simulink model "BMS_model_balancing"  (R2025b)
settings: Solver=FixedStepDiscrete  StartTime=0.0  StopTime=10  RelTol=1e-3
undefined symbols (not defined in the file): balanceResis, BalThreshold, chargeCurrent, currentLim, dischargeCurrent, initialSOC, stepTime, tempLim, Ts
libraries: fl_lib x128, nesl_utility x105, ee_lib x24, batteryecm_lib x24, simulink x5, BatteryBalancing x2, BatteryCurrentManagement x1
(part 1 of 5)
settings Model: Creator=Kevin  LastModifiedBy=kevpc
settings DataIOCC: ExternalInput=test_temp.getElement('Temp 1'),test_temp.getElement('Temp 2')  LoadExternalInput=on
settings OptimizationCC: DefaultParameterBehavior=Inlined  EnhancedBackFolding=on  PassReuseOutputArgsAs=Individual arguments  ZeroExternalMemoryAtStartup=off  ZeroInternalMemoryAtStartup=off  OptimizeBlockOrder=speed  DifferentSizesBufferReuse=on  OptimizationCustomize=off  EfficientTunableParamExpr=on
settings DebuggingCC: SolverPrmCheckMsg=warning  ParameterTunabilityLossMsg=error  StateNameClashWarn=warning
settings HardwareCC: ProdBitPerInt=16.0  ProdBitPerPointer=16.0  ProdBitPerSizeT=16.0  ProdBitPerPtrDiffT=16.0  ProdLargestAtomicFloat=None  ProdWordSize=16.0  ProdHWDeviceType=STMicroelectronics->ST10/Super10
settings SFSimCC: MATLABDynamicMemAlloc=off  SimTargetLang=C++  SimDLTargetLibrary=mkl-dnn
settings RTWCC: SystemTargetFile=ert.tlc  TemplateMakefile=ert_default_tmf  BuildConfiguration=Faster Runs  PortableWordSizes=on  DataTypeReplacement=CDataTypesFixedWidth  TargetLang=C++  GPUComputeCapability=3.5  Description=Embedded Coder
settings CodeAppCC: ForceParamTrailComments=on  IgnoreCustomStorageClasses=off  OperatorAnnotations=on  SimulinkDataObjDesc=on  SFDataObjDesc=on  MATLABFcnDesc=on  InsertBlockDesc=on  StateflowObjectComments=on  InlinedPrmAccess=Macros
settings ERTTargetCC: RootIOFormat=Structure reference  ERTCustomFileTemplate=example_file_process.tlc  ERTFilePackagingFormat=Compact  SuppressUnreachableDefaultCases=off  IndentSize=4  MaxIdInt64=INT64_MAX  MinIdInt64=INT64_MIN  MaxIdUint64=UINT64_MAX  MaxIdInt32=INT32_MAX  MinIdInt32=INT32_MIN  MaxIdUint32=UINT32_MAX  MaxIdInt16=INT16_MAX  MinIdInt16=INT16_MIN  MaxIdUint16=UINT16_MAX  MaxIdInt8=INT8_MAX  MinIdInt8=INT8_MIN  MaxIdUint8=UINT8_MAX  DynamicArrayContainerType=coder::array  TargetLangStandard=C++11 (ISO)  GenerateSampleERTMain=on  CodeInterfacePackaging=C++ class  SubcomponentCodeInterfacePackaging=C++ class  PurelyIntegerCode=on  SupportNonFinite=off  SupportComplex=off  CastingMode=Standards  ArrayLayout=Row-major

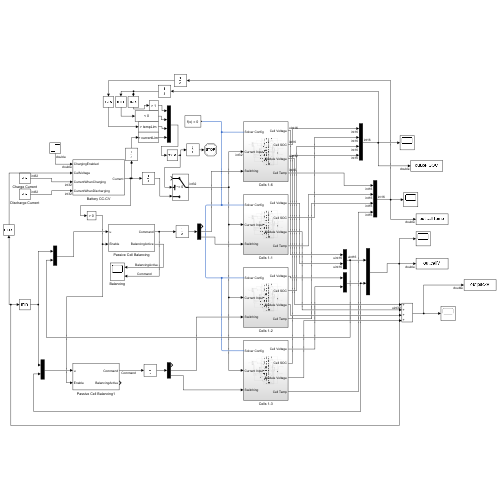
[thumbnail: Simulink's stored preview of the top-level diagram]
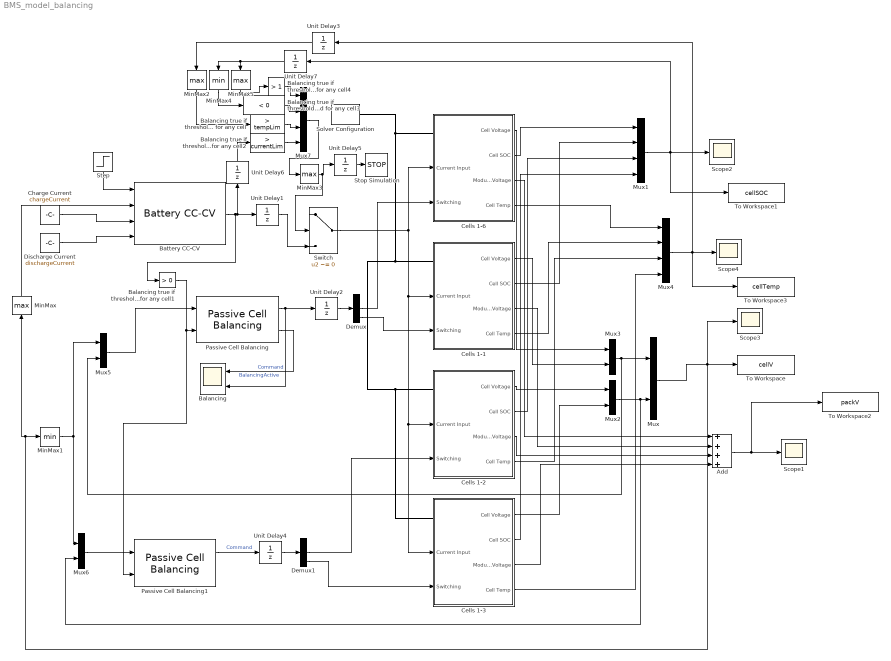
== system BMS_model_balancing ==
  Add : Sum  Inputs=++++
  Balancing : Scope  NumInputPorts=2
      settings: ActiveDisplayYMinimum=-1  ActiveDisplayYMaximum=1
  Balancing true if threshold exceeded for any cell : simulink/Logic and Bit Operations/Compare To Constant  relop=>  const=tempLim  OutDataTypeStr=boolean
  Balancing true if threshold exceeded for any cell1 : simulink/Logic and Bit Operations/Compare To Constant  relop=>  const=0  OutDataTypeStr=boolean
  Balancing true if threshold exceeded for any cell2 : simulink/Logic and Bit Operations/Compare To Constant  relop=>  const=currentLim  OutDataTypeStr=boolean
  Balancing true if threshold exceeded for any cell3 : simulink/Logic and Bit Operations/Compare To Constant  relop=<  const=0  OutDataTypeStr=boolean
  Balancing true if threshold exceeded for any cell4 : simulink/Logic and Bit Operations/Compare To Constant  relop=>  const=1  OutDataTypeStr=boolean
  Battery CC-CV : BatteryCurrentManagement/Battery CC-CV  MinMaxFlag=off  MaxCellVoltage=4.15  Kp=100  Ki=10  Kaw=1  Kt=1  Ts=Ts
      settings: LibrarySourceBlock=batt_sl_lib/Current Management/Battery CC-CV
  Cells 1-1 : Subsystem
      settings: PortSchema="{\"entries\":[{\"content\":{\"sides\":[{\"content\":{\"connectorIds\":[\"LConn1\",\"In1\",\"In2\"]},\"type\":\"ConnectorPlacement.EquallySpacedRectSide\",\"uuid\":\"db30e550-17cb-4259-84ee-fd9a91d57a68\"},{\"content\":{\"connectorIds\":[\"Out1\",\"Out2\",\"Out3\",\"Out4\"],\"side\":\"RIGHT\"},\"type\":\"ConnectorPlacement.EquallySpacedRectSide\",\"uuid\":\"cbb001cf-4149-4e45-8786-c11ff4e2edad\"},{\"content\":{\"side\":\"TOP\"},\"type\":\"ConnectorPlacement.EquallySpacedRectSide\",\"uuid\":\"46011520-7272-4d82-b54c-25ab64d6479d\"}]},\"type\":\"ConnectorPlacement.EquallySpacedConnector\",\"uuid\":\"f02d7cf1-4216-40a9-b502-774a48e892cb\"}],\"packageUris\":[\"http://schema.mathworks.com/mf0/Connector/R2020b\"],\"version\":\"1.0\"}"
  Cells 1-2 : Subsystem
      settings: PortSchema="{\"entries\":[{\"content\":{\"sides\":[{\"content\":{\"connectorIds\":[\"LConn1\",\"In1\",\"In2\"]},\"type\":\"ConnectorPlacement.EquallySpacedRectSide\",\"uuid\":\"db30e550-17cb-4259-84ee-fd9a91d57a68\"},{\"content\":{\"connectorIds\":[\"Out1\",\"Out2\",\"Out3\",\"Out4\"],\"side\":\"RIGHT\"},\"type\":\"ConnectorPlacement.EquallySpacedRectSide\",\"uuid\":\"cbb001cf-4149-4e45-8786-c11ff4e2edad\"},{\"content\":{\"side\":\"TOP\"},\"type\":\"ConnectorPlacement.EquallySpacedRectSide\",\"uuid\":\"46011520-7272-4d82-b54c-25ab64d6479d\"}]},\"type\":\"ConnectorPlacement.EquallySpacedConnector\",\"uuid\":\"f02d7cf1-4216-40a9-b502-774a48e892cb\"}],\"packageUris\":[\"http://schema.mathworks.com/mf0/Connector/R2020b\"],\"version\":\"1.0\"}"
  Cells 1-3 : Subsystem
      settings: PortSchema="{\"entries\":[{\"content\":{\"sides\":[{\"content\":{\"connectorIds\":[\"LConn1\",\"In1\",\"In2\"]},\"type\":\"ConnectorPlacement.EquallySpacedRectSide\",\"uuid\":\"db30e550-17cb-4259-84ee-fd9a91d57a68\"},{\"content\":{\"connectorIds\":[\"Out1\",\"Out2\",\"Out3\",\"Out4\"],\"side\":\"RIGHT\"},\"type\":\"ConnectorPlacement.EquallySpacedRectSide\",\"uuid\":\"cbb001cf-4149-4e45-8786-c11ff4e2edad\"},{\"content\":{\"side\":\"TOP\"},\"type\":\"ConnectorPlacement.EquallySpacedRectSide\",\"uuid\":\"46011520-7272-4d82-b54c-25ab64d6479d\"}]},\"type\":\"ConnectorPlacement.EquallySpacedConnector\",\"uuid\":\"f02d7cf1-4216-40a9-b502-774a48e892cb\"}],\"packageUris\":[\"http://schema.mathworks.com/mf0/Connector/R2020b\"],\"version\":\"1.0\"}"
  Cells 1-6 : Subsystem
      settings: PortSchema="{\"entries\":[{\"content\":{\"sides\":[{\"content\":{\"connectorIds\":[\"LConn1\",\"In1\",\"In2\"]},\"type\":\"ConnectorPlacement.EquallySpacedRectSide\",\"uuid\":\"db30e550-17cb-4259-84ee-fd9a91d57a68\"},{\"content\":{\"connectorIds\":[\"Out1\",\"Out2\",\"Out3\",\"Out4\"],\"side\":\"RIGHT\"},\"type\":\"ConnectorPlacement.EquallySpacedRectSide\",\"uuid\":\"cbb001cf-4149-4e45-8786-c11ff4e2edad\"},{\"content\":{\"side\":\"TOP\"},\"type\":\"ConnectorPlacement.EquallySpacedRectSide\",\"uuid\":\"46011520-7272-4d82-b54c-25ab64d6479d\"}]},\"type\":\"ConnectorPlacement.EquallySpacedConnector\",\"uuid\":\"f02d7cf1-4216-40a9-b502-774a48e892cb\"}],\"packageUris\":[\"http://schema.mathworks.com/mf0/Connector/R2020b\"],\"version\":\"1.0\"}"
  Charge Current : Constant  Value=chargeCurrent  OutDataTypeStr=int32
  Demux : Demux  Outputs=[1, 6, 6]
  Demux1 : Demux  Outputs=[1, 6, 6]
  Discharge Current : Constant  Value=dischargeCurrent  OutDataTypeStr=int32
  MinMax{,2..3,5} (4 alike) : MinMax  Function=max
  MinMax1 : MinMax
  MinMax4 : MinMax
  Mux{,2..3,5..6} (5 alike) : Mux  Inputs=2
  Mux1 : Mux
  Mux4 : Mux
  Mux7 : Mux
  Passive Cell Balancing : BatteryBalancing/Passive Cell Balancing  Threshold=BalThreshold  HysteresisBand=0  Td_on=1  Td_off=1  Ts=Ts  dataType=double
      settings: LibrarySourceBlock=batt_sl_lib/Cell Balancing/Passive Cell Balancing
  Passive Cell Balancing1 : BatteryBalancing/Passive Cell Balancing  Threshold=BalThreshold  HysteresisBand=0  Td_on=1  Td_off=1  Ts=Ts  dataType=double
      settings: LibrarySourceBlock=batt_sl_lib/Cell Balancing/Passive Cell Balancing
  Scope{1..4} (4 alike) : Scope
      Scope1 settings: ActiveDisplayYMinimum=-1  ActiveDisplayYMaximum=1
      Scope2 settings: ActiveDisplayYMinimum=0.17993293226878598  ActiveDisplayYMaximum=1.01289263881682
      Scope3 settings: ActiveDisplayYMinimum=3.8472771421151224  ActiveDisplayYMaximum=5.4386775854572109  DataLoggingVariableName=ScopeData2
      Scope4 settings: ActiveDisplayYMinimum=-1  ActiveDisplayYMaximum=1  DataLoggingVariableName=ScopeData3
  Solver Configuration : nesl_utility/Solver Configuration  PhysicalDomain=network_engine_domain  SubClassName=solver  LeftPortType=input  RightPortType=generic  Tones=[]  Harmonics=[]  SimulateNoise=off  Profile=off  UseLocalSampling=off  EnableSwitchedLinearOptims=on  FrequencyDomain=off  UseCCode=off  RelTol=0.001  AbsTol=0.001  MinStep=1e-09  ToWorkspace=off  RevertToSquareIcSolve=off  NumHomotopyIterations=100  PhasorMode=off  PhasorModeNumHarmonics=1  ConsistencySolver=NEWTON_XTOL_AFTER_FTOL  IndexReductionMethod=DerivativeReplacement  DoDC=off  ResidualTolerance=1e-09  ConsistencyTolSource=GLOBAL  ConsistencyAbsTol=0.001  ConsistencyRelTol=0.001  ConsistencyTolFactor=0.001  UseLocalSolver=on  LocalSolverChoice=NE_BACKWARD_EULER_ADVANCER  ResolveIndetEquations=on  FunctionEvalNumThread=1  LocalSolverSampleTime=Ts  DoFixedCost=on  MaxNonlinIter=3  MaxModeIter=2  ComputeImpulses=off  ImpulseIterations=2  LinearAlgebra=auto  LinearAlgebraNumThread=0  EquationFormulation=NE_TIME_EF  DelaysMemoryBudget=1024  AutomaticFiltering=on  FilteringTimeConstant=0.001  PartitionStorageMethod=AS_NEEDED  PartitionMemoryBudget=1024  PartitionMethod=ROBUST  MultibodyUseLocalSolver=off  MultibodyLocalSolverChoice=ODE1  MultibodyLocalSolverSampleTime=0.001
  Step : Step  Time=stepTime  SampleTime=1
  Stop Simulation : Stop
  Switch : Switch  Criteria=u2 ~= 0  SaturateOnIntegerOverflow=off  InputSameDT=off
  To Workspace : ToWorkspace  VariableName=cellV  SampleTime=-1
      settings: Save2DSignal=2-D array (concatenate along first dimension)
  To Workspace1 : ToWorkspace  VariableName=cellSOC  SampleTime=-1
      settings: Save2DSignal=2-D array (concatenate along first dimension)
  To Workspace2 : ToWorkspace  VariableName=packV  SaveFormat=Timeseries  SampleTime=-1
  To Workspace3 : ToWorkspace  VariableName=cellTemp  SampleTime=-1
      settings: Save2DSignal=2-D array (concatenate along first dimension)
  Unit Delay{1..7} (7 alike) : UnitDelay  SampleTime=-1  HasFrameUpgradeWarning=on
  wires:
  Step/1 -> Battery CC-CV/1
  Passive Cell Balancing/1 -> Balancing/2, Unit Delay2/1  "Command"
  Battery CC-CV/1 -> Unit Delay1/1, Unit Delay6/1, Balancing true if threshold exceeded for any cell1/1
  Balancing true if threshold exceeded for any cell1/1 -> Passive Cell Balancing1/2, Passive Cell Balancing/2
  Charge Current/1 -> Battery CC-CV/3
  Add/1 -> To Workspace2/1, Scope1/1
  Passive Cell Balancing/2 -> Balancing/1  "BalancingActive"
  Switch/1 -> Cells 1-6/1(Current Input), Cells 1-1/1(Current Input), Cells 1-3/1(Current Input), Cells 1-2/1(Current Input)
  Mux/1 -> Scope3/1, MinMax1/1, MinMax/1, To Workspace/1
  Mux1/1 -> Unit Delay7/1, To Workspace1/1, Scope2/1
  Cells 1-6/2(Cell SOC) -> Mux1/1
  Cells 1-1/2(Cell SOC) -> Mux1/2
  Cells 1-2/2(Cell SOC) -> Mux1/3
  Cells 1-3/2(Cell SOC) -> Mux1/4
  Unit Delay2/1 -> Demux/1
  Demux/2 -> Cells 1-6/2(Switching)
  Demux/3 -> Cells 1-1/2(Switching)
  Passive Cell Balancing1/1 -> Unit Delay4/1  "Command"
  Unit Delay4/1 -> Demux1/1
  Demux1/2 -> Cells 1-2/2(Switching)
  Demux1/3 -> Cells 1-3/2(Switching)
  Mux3/1 -> Mux5/2, Mux/1
  Mux2/1 -> Mux6/2, Mux/2
  Cells 1-3/1(Cell Voltage) -> Mux2/2
  Cells 1-2/1(Cell Voltage) -> Mux2/1
  Cells 1-1/1(Cell Voltage) -> Mux3/2
  Cells 1-6/1(Cell Voltage) -> Mux3/1
  Cells 1-6/3(Module Voltage) -> Add/1
  Cells 1-1/3(Module Voltage) -> Add/2
  Cells 1-2/3(Module Voltage) -> Add/3
  Cells 1-3/3(Module Voltage) -> Add/4
  MinMax/1 -> Battery CC-CV/2
  Cells 1-6/4(Cell Temp) -> Mux4/1
  Cells 1-1/4(Cell Temp) -> Mux4/2
  Cells 1-2/4(Cell Temp) -> Mux4/3
  Cells 1-3/4(Cell Temp) -> Mux4/4
  Mux4/1 -> Unit Delay3/1, To Workspace3/1, Scope4/1
  Mux5/1 -> Passive Cell Balancing/1
  Mux6/1 -> Passive Cell Balancing1/1
  MinMax1/1 -> Mux6/1, Mux5/1
  Unit Delay1/1 -> Switch/3
  MinMax2/1 -> Balancing true if threshold exceeded for any cell/1
  Unit Delay3/1 -> MinMax2/1
  Discharge Current/1 -> Battery CC-CV/4
  Unit Delay5/1 -> Stop Simulation/1
  Balancing true if threshold exceeded for any cell2/1 -> Mux7/4
  Balancing true if threshold exceeded for any cell/1 -> Mux7/3
  MinMax3/1 -> Switch/2, Unit Delay5/1
  Mux7/1 -> MinMax3/1
  Unit Delay6/1 -> Balancing true if threshold exceeded for any cell2/1
  Balancing true if threshold exceeded for any cell3/1 -> Mux7/2
  MinMax4/1 -> Balancing true if threshold exceeded for any cell3/1
  Unit Delay7/1 -> MinMax5/1, MinMax4/1
  MinMax5/1 -> Balancing true if threshold exceeded for any cell4/1
  Balancing true if threshold exceeded for any cell4/1 -> Mux7/1
  connections:
  Solver Configuration/RConn1 -- Cells 1-1/LConn1 -- Cells 1-3/LConn1 -- Cells 1-2/LConn1 -- Cells 1-6/LConn1
